simulink model "Question_2"  (R2024b)
settings: Solver=VariableStepAuto  StartTime=0.0  StopTime=10.0  RelTol=1e-3
model workspace (MAT data in the model file):
  I = 0.088
  L = 0.43
  g = 9.81
  m = 1
settings Model: Creator=Sagar  LastModifiedBy=Sagar

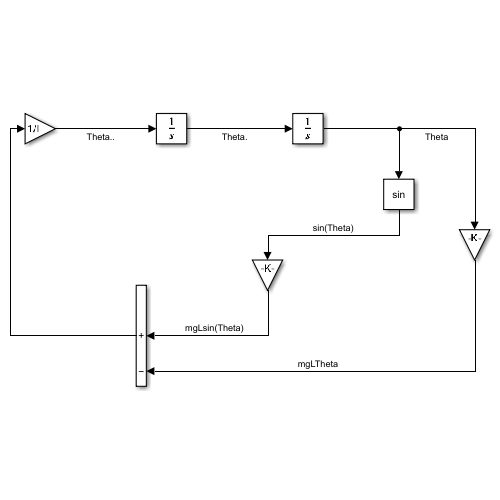
[thumbnail: Simulink's stored preview of the top-level diagram]
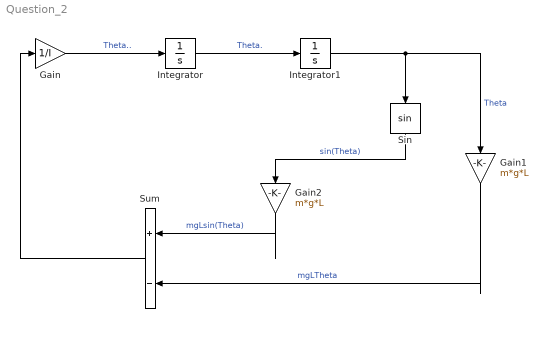
== system Question_2 ==
  Gain : Gain  Gain=1/I
  Gain1 : Gain  Gain=m*g*L
  Gain2 : Gain  Gain=m*g*L
  Integrator : Integrator
  Integrator1 : Integrator
  Sin : Trigonometry
  Sum : Sum  Inputs=|+-
  wires:
  Gain/1 -> Integrator/1  "Theta.."
  Integrator/1 -> Integrator1/1  "Theta."
  Sum/1 -> Gain/1
  Integrator1/1 -> Sin/1, Gain1/1  "Theta"
  Gain1/1 -> Sum/2  "mgLTheta"
  Sin/1 -> Gain2/1  "sin(Theta)"
  Gain2/1 -> Sum/1  "mgLsin(Theta)"
